simulink model "FloatingBall"  (R2024b)
settings: Solver=FixedStepAuto  StartTime=0.0  StopTime=inf  RelTol=1e-3  EnableMultiTasking=on
undefined symbols (not defined in the file or in its folder): Start
libraries: arduinolib x10, arduinoavrlib x2
settings Model: ExtModeTrigDuration=2  Creator=Tim  LastModifiedBy=Alexander
settings SolverCC: AutoInsertRateTranBlk=on
settings OptimizationCC: DefaultParameterBehavior=Inlined  EnhancedBackFolding=on  PassReuseOutputArgsAs=Individual arguments  ZeroExternalMemoryAtStartup=off  ZeroInternalMemoryAtStartup=off  MaxStackSize=64  OptimizeBlockOrder=speed  DifferentSizesBufferReuse=on  OptimizationCustomize=off  EfficientTunableParamExpr=on
settings DebuggingCC: MultiTaskDSMMsg=none  ParameterTunabilityLossMsg=error
settings HardwareCC: ProdBitPerInt=16  ProdBitPerPointer=16  ProdBitPerSizeT=16  ProdBitPerPtrDiffT=16  ProdLargestAtomicFloat=None  ProdWordSize=8  ProdHWDeviceType=Atmel->AVR
settings SFSimCC: MATLABDynamicMemAlloc=off
settings RTWCC: Description=Embedded Coder  SystemTargetFile=ert.tlc  HardwareBoard=Arduino Uno  TemplateMakefile=ert_default_tmf  Toolchain=Arduino AVR  BuildConfiguration=Faster Runs
settings CodeAppCC: ForceParamTrailComments=on  IgnoreCustomStorageClasses=off  OperatorAnnotations=on  SimulinkDataObjDesc=on  SFDataObjDesc=on  InsertBlockDesc=on
settings ERTTargetCC: SupportContinuousTime=on  SupportVariableSizeSignals=on  ExtModeTransport=3  ExtModeStaticAlloc=on  ExtModeAutomaticAllocSize=off  ExtModeStaticAllocSize=250  ExtModeMexFile=ext_xcp  ExtModeIntrfLevel=Level2 - Open

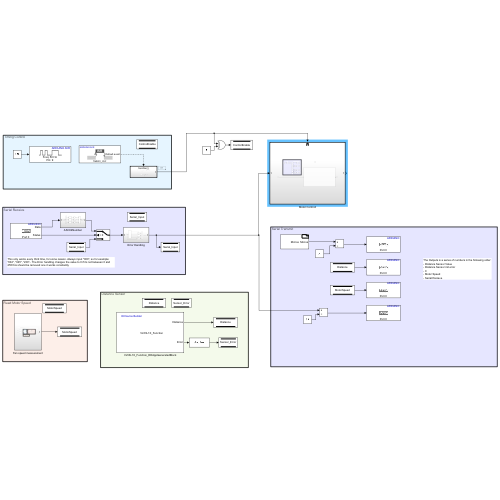
[thumbnail: Simulink's stored preview of the top-level diagram]
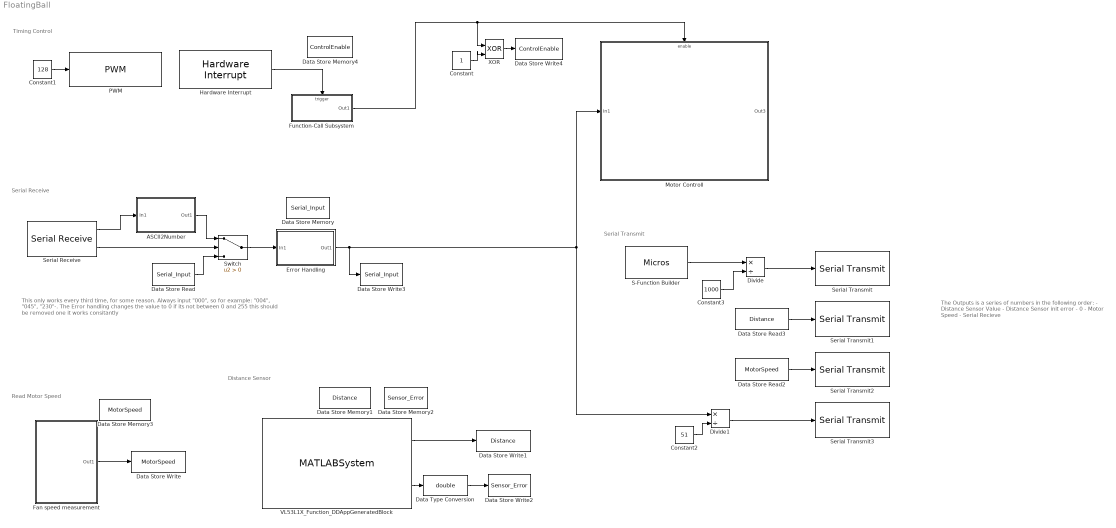
== system FloatingBall ==
  note: Timing Control
  note: Serial Receive
  note: This only works every third time, for some reason. Always input "000", so for example: "004", "045", "230"-. The Error handling changes the value to 0 if its not between 0 and 255 this should be removed one it works consitantly
  note: Read Motor Speed
  note: Distance Sensor
  note: The Outputs is a series of numbers in the following order:
      | - Distance Sensor Value
      | - Distance Sensor init error
      | - 0
      | - Motor Speed
      | - Serial Recieve
  note: Serial Transmit
  ASCII2Number : Subsystem
  Constant : Constant
  Constant1 : Constant  Value=128
  Constant2 : Constant  Value=51
  Constant3 : Constant  Value=1000
  Data Store Memory : DataStoreMemory  DataStoreName=Serial_Input  WriteAfterWriteMsg=warning  ShowAdditionalParam=off
  Data Store Memory1 : DataStoreMemory  DataStoreName=Distance  WriteAfterWriteMsg=warning  ShowAdditionalParam=off
  Data Store Memory2 : DataStoreMemory  DataStoreName=Sensor_Error  WriteAfterWriteMsg=warning  ShowAdditionalParam=off
  Data Store Memory3 : DataStoreMemory  DataStoreName=MotorSpeed  WriteAfterWriteMsg=warning  ShowAdditionalParam=off
  Data Store Memory4 : DataStoreMemory  DataStoreName=ControlEnable  WriteAfterWriteMsg=warning  ShowAdditionalParam=off
  Data Store Read : DataStoreRead  DataStoreName=Serial_Input  IndexOptions=Index vector (dialog)  Indices=1  OutputSizes=1
  Data Store Read2 : DataStoreRead  DataStoreName=MotorSpeed  IndexOptions=Index vector (dialog)  Indices=1  OutputSizes=1
  Data Store Read3 : DataStoreRead  DataStoreName=Distance  IndexOptions=Index vector (dialog)  Indices=1  OutputSizes=1
  Data Store Write : DataStoreWrite  DataStoreName=MotorSpeed  IndexOptions=Index vector (dialog)  Indices=1  OutputSizes=1
  Data Store Write1 : DataStoreWrite  DataStoreName=Distance  IndexOptions=Index vector (dialog)  Indices=1  OutputSizes=1
  Data Store Write2 : DataStoreWrite  DataStoreName=Sensor_Error  IndexOptions=Index vector (dialog)  Indices=1  OutputSizes=1
  Data Store Write3 : DataStoreWrite  DataStoreName=Serial_Input  IndexOptions=Index vector (dialog)  Indices=1  OutputSizes=1
  Data Store Write4 : DataStoreWrite  DataStoreName=ControlEnable  IndexOptions=Index vector (dialog)  Indices=1  OutputSizes=1
  Data Type Conversion : DataTypeConversion  OutDataTypeStr=double  SaturateOnIntegerOverflow=off  RndMeth=Floor
  Divide : Product  Inputs=*/
  Divide1 : Product  Inputs=*/
  Error Handling : Subsystem
  Fan speed measurement : Subsystem
  Function-Call Subsystem : Subsystem  TreatAsAtomicUnit=on
  Hardware Interrupt : arduinoavrlib/Hardware Interrupt  ISRGroup=Timer 1  ISRName=TIMER1_OVF  ISRNumber=7  EventsList={'on','Default event','1'}  SelectedEvents={'Default event'}  TaskPriority=8  DisablePreemption=on  ClearInterruptFlagsAtEndOfEvent=off  HardwareBoard=ARDUINO AVR
  Motor Controll : Subsystem
  PWM : arduinoavrlib/PWM  pinNumber=9  desiredFrequency=50  achievableFrequency=50  EnableCompareMatchInterrupt=off  EnableOverflowInterrupt=on
  S-Function Builder : S-Function  FunctionName=Micros  SFunctionModules=Micros_wrapper.c  SFunctionDeploymentMode=off  EnableBusSupport=off  mask(S-Function Builder){}
      mask help: Simulink:masks:SFunctionBuilder_MD
      mask init:
      | val = [[.9  0.75 0.75 1 1 .9 .9 1]',[1 1 0.75 0.75 .9 .9 1 .9]'];try , sys = get_param(gcb,'SfunBuilderFcnName');if isempty(sys), sys = get_param(gcb,'FunctionName'); end,catch, sys = get_param(gcb,'FunctionName'); end
      settings: CopyFcn=set_param(gcbh,'LinkStatus','none')  OpenFcn=sfunctionwizard(gcbh)
      mask Display:
      | plot(val(:,1),val(:,2))
      | disp(sys)
      | port_label('output',1,sprintf('%s', 'Micros'),'interpreter','tex')
  Serial Receive : arduinolib/Serial Receive  portNumber=0  DataType=uint8  blockPlatform=ARDUINO  TimeOut=0  MaxDataLength=2  isARMArch=off  DataLengthOption=Length via dialog  Datalength=3  Header=[]  Terminator=[]  SampleTime=0.02  ShowOutStatus=on
  Serial Transmit : arduinolib/Serial Transmit  portNumber=0  sendmode=print  label=;Start:  sendformat=Decimal  floatprecision=2  header=[]  terminator=[]  blockPlatform=ARDUINO
  Serial Transmit1 : arduinolib/Serial Transmit  portNumber=0  sendmode=print  label=;  sendformat=Decimal  floatprecision=1  header=[]  terminator=[]  blockPlatform=ARDUINO
  Serial Transmit2 : arduinolib/Serial Transmit  portNumber=0  sendmode=print  label=;  sendformat=Decimal  floatprecision=1  header=[]  terminator=[]  blockPlatform=ARDUINO
  Serial Transmit3 : arduinolib/Serial Transmit  portNumber=0  sendmode=print  label=;  sendformat=Decimal  floatprecision=2  header=[]  terminator=[]  blockPlatform=ARDUINO
  Switch : Switch  Criteria=u2 > Threshold  SaturateOnIntegerOverflow=off  InputSameDT=off
  VL53L1X_Function_DDAppGeneratedBlock : MATLABSystem  System=VL53L1X_Function  SampleTime=0.02
      mask Type: VL53L1X_Function
      mask Display:
      | color('white');plot([100,100,100,100]*1,[100,100,100,100]*1);plot([100,100,100,100]*0,[100,100,100,100]*0);color('blue');text(38, 92, 'IO Device Builder','horizontalAlignment', 'right');
      | color('black');text(52,50,' VL53L1X_Function','horizontalAlignment','center');
      | port_label('output',1,'Distance');port_label('output',2,'Error');
  XOR : Logic  Operator=XOR  IconShape=distinctive  AllPortsSameDT=off  OutDataTypeStr=boolean
  wires:
  Serial Receive/2 -> Switch/2
  Data Store Read/1 -> Switch/3
  Serial Receive/1 -> ASCII2Number/1(In1)
  ASCII2Number/1(Out1) -> Switch/1
  Switch/1 -> Error Handling/1(In1)
  Constant1/1 -> PWM/1
  Hardware Interrupt/1 -> Function-Call Subsystem/Trigger
  Fan speed measurement/1(Out1) -> Data Store Write/1
  VL53L1X_Function_DDAppGeneratedBlock/1 -> Data Store Write1/1
  VL53L1X_Function_DDAppGeneratedBlock/2 -> Data Type Conversion/1
  Data Type Conversion/1 -> Data Store Write2/1
  Function-Call Subsystem/1(Out1) -> Motor Controll/Enable, XOR/1
  Data Store Read2/1 -> Serial Transmit2/1
  Data Store Read3/1 -> Serial Transmit1/1
  S-Function Builder/1 -> Divide/1
  Constant3/1 -> Divide/2
  Divide/1 -> Serial Transmit/1
  Constant2/1 -> Divide1/2
  Divide1/1 -> Serial Transmit3/1
  Error Handling/1(Out1) -> Divide1/1, Motor Controll/1(In1), Data Store Write3/1
  XOR/1 -> Data Store Write4/1
  Constant/1 -> XOR/2

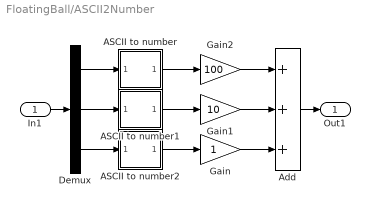
== system FloatingBall/ASCII2Number ==
  In1 : Inport
  ASCII to number : Subsystem
  ASCII to number1 : Subsystem
  ASCII to number2 : Subsystem
  Add : Sum  Inputs=+++
  Demux : Demux  Outputs=3
  Gain : Gain
  Gain1 : Gain  Gain=10
  Gain2 : Gain  Gain=100
  Out1 : Outport
  wires:
  Gain1/1 -> Add/2
  Gain2/1 -> Add/1
  Gain/1 -> Add/3
  Demux/1 -> ASCII to number/1(In1)
  ASCII to number2/1(Out1) -> Gain/1
  Demux/3 -> ASCII to number2/1(In1)
  ASCII to number/1(Out1) -> Gain2/1
  Demux/2 -> ASCII to number1/1(In1)
  ASCII to number1/1(Out1) -> Gain1/1
  Add/1 -> Out1/1
  In1/1 -> Demux/1

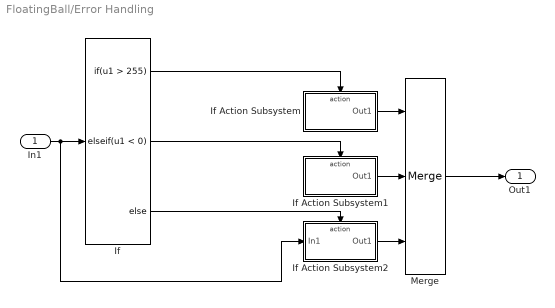
== system FloatingBall/Error Handling ==
  In1 : Inport
  If : If  IfExpression=u1 > 255  ElseIfExpressions=u1 < 0
  If Action Subsystem : Subsystem  TreatAsAtomicUnit=on
  If Action Subsystem1 : Subsystem  TreatAsAtomicUnit=on
  If Action Subsystem2 : Subsystem  TreatAsAtomicUnit=on
  Merge : Merge  Inputs=3
  Out1 : Outport
  wires:
  In1/1 -> If Action Subsystem2/1(In1), If/1
  If/1 -> If Action Subsystem/Action
  If/2 -> If Action Subsystem1/Action
  If/3 -> If Action Subsystem2/Action
  If Action Subsystem2/1(Out1) -> Merge/3
  If Action Subsystem1/1(Out1) -> Merge/2
  If Action Subsystem/1(Out1) -> Merge/1
  Merge/1 -> Out1/1

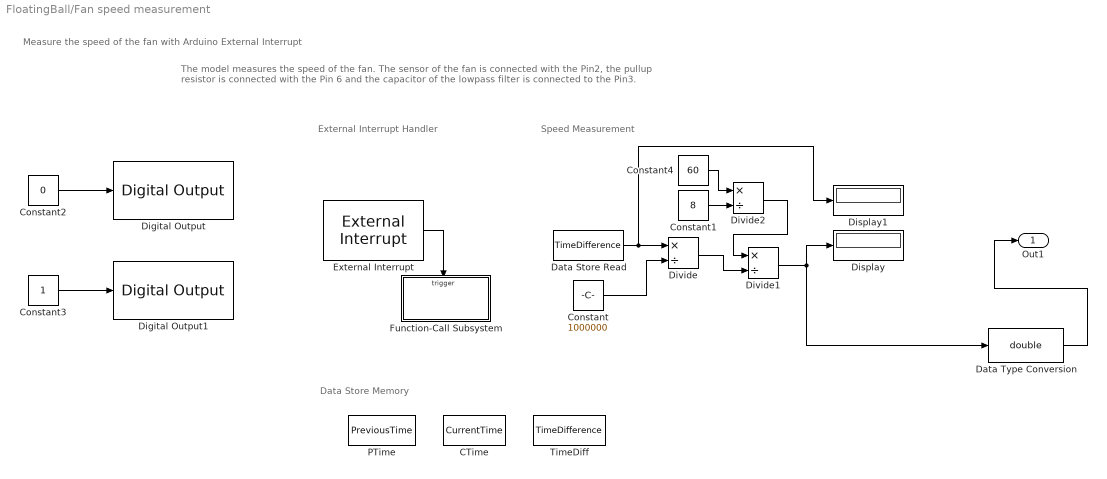
== system FloatingBall/Fan speed measurement ==
  note: External Interrupt Handler
  note: Speed Measurement
  note: Data Store Memory
  note: Measure the speed of the fan with Arduino External Interrupt
  note: The model measures the speed of the fan.
      | The sensor of the fan is connected with the Pin2, the pullup resistor is connected with the Pin 6 and
      | the capacitor of the lowpass filter is connected to the Pin3.
  CTime : DataStoreMemory  DataStoreName=CurrentTime  ShowAdditionalParam=off  OutDataTypeStr=uint32
  Constant : Constant  Value=1000000
  Constant1 : Constant  Value=8
  Constant2 : Constant  Value=0
  Constant3 : Constant
  Constant4 : Constant  Value=60
  Data Store Read : DataStoreRead  DataStoreName=TimeDifference  IndexOptions=Index vector (dialog)  Indices=1  OutputSizes=1
  Data Type Conversion : DataTypeConversion  OutDataTypeStr=double  SaturateOnIntegerOverflow=off  RndMeth=Floor
  Digital Output : arduinolib/Digital Output  pinNumber=3  Direction=output  blockPlatform=arduino
  Digital Output1 : arduinolib/Digital Output  pinNumber=6  Direction=output  blockPlatform=arduino
  Display : Display
  Display1 : Display
  Divide : Product  Inputs=*/
  Divide1 : Product  Inputs=*/
  Divide2 : Product  Inputs=*/
  External Interrupt : arduinolib/External Interrupt  Pin=2  PullUp=off  Mode=FALLING  InterruptSimulationInput=off
  Function-Call Subsystem : Subsystem  TreatAsAtomicUnit=on
  PTime : DataStoreMemory  DataStoreName=PreviousTime  ShowAdditionalParam=off  OutDataTypeStr=uint32
  TimeDiff : DataStoreMemory  DataStoreName=TimeDifference  ShowAdditionalParam=off  OutDataTypeStr=uint32
  Out1 : Outport
  wires:
  Divide/1 -> Divide1/2
  Constant/1 -> Divide/2
  External Interrupt/1 -> Function-Call Subsystem/Trigger
  Constant1/1 -> Divide2/2
  Data Store Read/1 -> Display1/1, Divide/1
  Constant3/1 -> Digital Output1/1
  Constant2/1 -> Digital Output/1
  Constant4/1 -> Divide2/1
  Data Type Conversion/1 -> Out1/1
  Divide2/1 -> Divide1/1
  Divide1/1 -> Display/1, Data Type Conversion/1

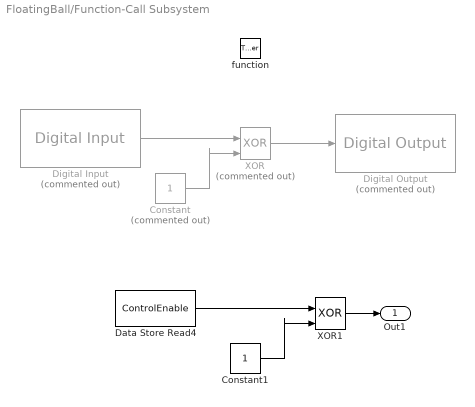
== system FloatingBall/Function-Call Subsystem ==
  function : TriggerPort  TriggerType=function-call  VariantControl=(inherit)
  Constant : Constant  Commented=on
  Constant1 : Constant
  Data Store Read4 : DataStoreRead  DataStoreName=ControlEnable  IndexOptions=Index vector (dialog)  Indices=1  OutputSizes=1
  Digital Input : arduinolib/Digital Input  Commented=on  pinNumber=12  mode=Default  Direction=input  SampleTime=-1  blockPlatform=arduino
  Digital Output : arduinolib/Digital Output  Commented=on  pinNumber=13  Direction=output  blockPlatform=arduino
  XOR : Logic  Commented=on  Operator=XOR  IconShape=distinctive  AllPortsSameDT=off  OutDataTypeStr=boolean
  XOR1 : Logic  Operator=XOR  IconShape=distinctive  AllPortsSameDT=off  OutDataTypeStr=boolean
  Out1 : Outport
  wires:
  Constant/1 -> XOR/2
  Digital Input/1 -> XOR/1
  XOR/1 -> Digital Output/1
  Constant1/1 -> XOR1/2
  Data Store Read4/1 -> XOR1/1
  XOR1/1 -> Out1/1

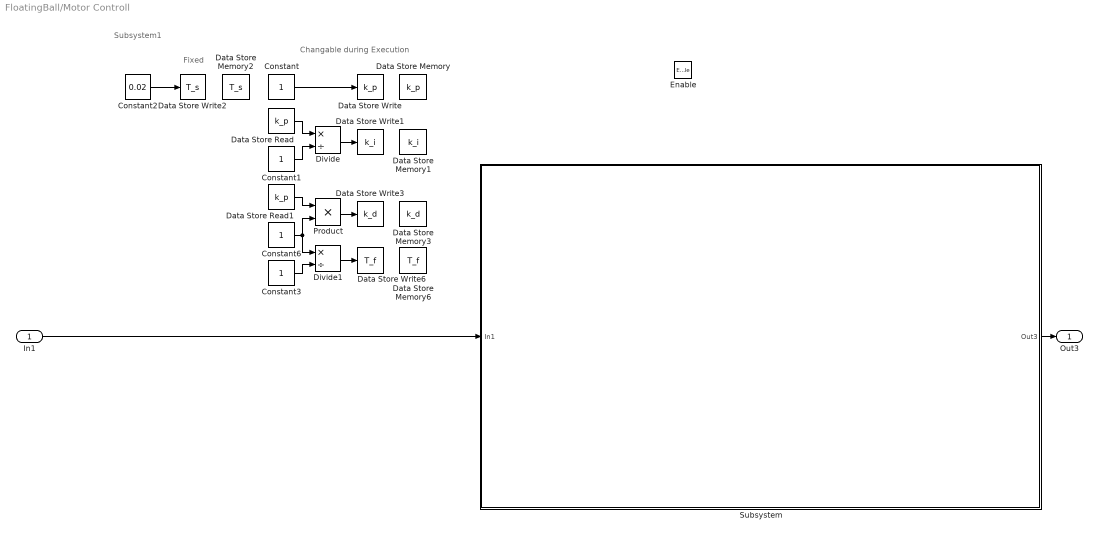
== system FloatingBall/Motor Controll ==
  note: Subsystem1
  note: Fixed
  note: Changable during Execution
  In1 : Inport
  Enable : EnablePort
  Constant{,1,3,6} (4 alike) : Constant
  Constant2 : Constant  Value=0.02
  Data Store Memory : DataStoreMemory  DataStoreName=k_p  WriteAfterWriteMsg=warning  ShowAdditionalParam=off
  Data Store Memory1 : DataStoreMemory  DataStoreName=k_i  WriteAfterWriteMsg=warning  ShowAdditionalParam=off
  Data Store Memory2 : DataStoreMemory  DataStoreName=T_s  WriteAfterWriteMsg=warning  ShowAdditionalParam=off
  Data Store Memory3 : DataStoreMemory  DataStoreName=k_d  WriteAfterWriteMsg=warning  ShowAdditionalParam=off
  Data Store Memory6 : DataStoreMemory  DataStoreName=T_f  WriteAfterWriteMsg=warning  ShowAdditionalParam=off
  Data Store Read : DataStoreRead  DataStoreName=k_p  IndexOptions=Index vector (dialog)  Indices=1  OutputSizes=1
  Data Store Read1 : DataStoreRead  DataStoreName=k_p  IndexOptions=Index vector (dialog)  Indices=1  OutputSizes=1
  Data Store Write : DataStoreWrite  DataStoreName=k_p  IndexOptions=Index vector (dialog)  Indices=1  OutputSizes=1
  Data Store Write1 : DataStoreWrite  DataStoreName=k_i  IndexOptions=Index vector (dialog)  Indices=1  OutputSizes=1
  Data Store Write2 : DataStoreWrite  DataStoreName=T_s  IndexOptions=Index vector (dialog)  Indices=1  OutputSizes=1
  Data Store Write3 : DataStoreWrite  DataStoreName=k_d  IndexOptions=Index vector (dialog)  Indices=1  OutputSizes=1
  Data Store Write6 : DataStoreWrite  DataStoreName=T_f  IndexOptions=Index vector (dialog)  Indices=1  OutputSizes=1
  Divide : Product  Inputs=*/
  Divide1 : Product  Inputs=*/
  Product : Product
  Subsystem : Subsystem
  Out3 : Outport
  wires:
  In1/1 -> Subsystem/1(In1)
  Subsystem/1(Out3) -> Out3/1
  Divide/1 -> Data Store Write1/1
  Data Store Read1/1 -> Product/1
  Data Store Read/1 -> Divide/1
  Product/1 -> Data Store Write3/1
  Constant2/1 -> Data Store Write2/1
  Constant1/1 -> Divide/2
  Constant/1 -> Data Store Write/1
  Divide1/1 -> Data Store Write6/1
  Constant3/1 -> Divide1/2
  Constant6/1 -> Divide1/1, Product/2

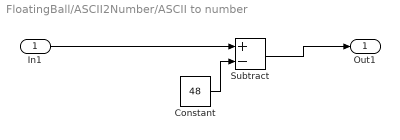
== system FloatingBall/ASCII2Number/ASCII to number ==
  In1 : Inport
  Constant : Constant  Value=48
  Subtract : Sum  Inputs=+-
  Out1 : Outport
  wires:
  In1/1 -> Subtract/1
  Constant/1 -> Subtract/2
  Subtract/1 -> Out1/1

== system FloatingBall/ASCII2Number/ASCII to number1 ==
  In1 : Inport
  Constant : Constant  Value=48
  Subtract : Sum  Inputs=+-
  Out1 : Outport
  wires:
  In1/1 -> Subtract/1
  Constant/1 -> Subtract/2
  Subtract/1 -> Out1/1

== system FloatingBall/ASCII2Number/ASCII to number2 ==
  In1 : Inport
  Constant : Constant  Value=48
  Subtract : Sum  Inputs=+-
  Out1 : Outport
  wires:
  In1/1 -> Subtract/1
  Constant/1 -> Subtract/2
  Subtract/1 -> Out1/1

== system FloatingBall/Error Handling/If Action Subsystem ==
  Action Port : ActionPort  ActionPortLabel=if(u1 > 255)
  Constant : Constant  Value=0
  Out1 : Outport
  wires:
  Constant/1 -> Out1/1

== system FloatingBall/Error Handling/If Action Subsystem1 ==
  Action Port : ActionPort  ActionPortLabel=elseif(u1 < 0)
  Constant : Constant  Value=0
  Out1 : Outport
  wires:
  Constant/1 -> Out1/1

== system FloatingBall/Error Handling/If Action Subsystem2 ==
  In1 : Inport
  Action Port : ActionPort  ActionPortLabel=else
  Out1 : Outport
  wires:
  In1/1 -> Out1/1

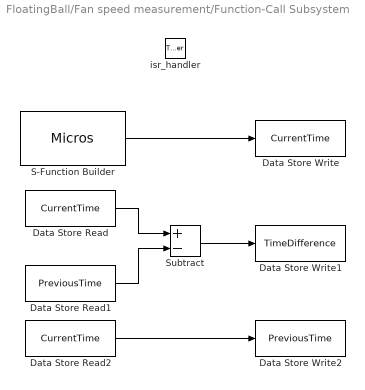
== system FloatingBall/Fan speed measurement/Function-Call Subsystem ==
  isr_handler : TriggerPort  TriggerType=function-call  VariantControl=Variant
  Data Store Read : DataStoreRead  DataStoreName=CurrentTime  IndexOptions=Index vector (dialog)  Indices=1  OutputSizes=1
  Data Store Read1 : DataStoreRead  DataStoreName=PreviousTime  IndexOptions=Index vector (dialog)  Indices=1  OutputSizes=1
  Data Store Read2 : DataStoreRead  DataStoreName=CurrentTime  IndexOptions=Index vector (dialog)  Indices=1  OutputSizes=1
  Data Store Write : DataStoreWrite  Priority=1  DataStoreName=CurrentTime  IndexOptions=Index vector (dialog)  Indices=1  OutputSizes=1
  Data Store Write1 : DataStoreWrite  Priority=2  DataStoreName=TimeDifference  IndexOptions=Index vector (dialog)  Indices=1  OutputSizes=1
  Data Store Write2 : DataStoreWrite  Priority=3  DataStoreName=PreviousTime  IndexOptions=Index vector (dialog)  Indices=1  OutputSizes=1
  S-Function Builder : S-Function  FunctionName=Micros  SFunctionModules=Micros_wrapper.c  SFunctionDeploymentMode=off  EnableBusSupport=off  mask(S-Function Builder){}
      mask help: Simulink:masks:SFunctionBuilder_MD
      mask init: same as FloatingBall/S-Function Builder
      settings: CopyFcn=set_param(gcbh,'LinkStatus','none')  OpenFcn=sfunctionwizard(gcbh)
      mask Display:
      | plot(val(:,1),val(:,2))
      | disp(sys)
      | port_label('output',1,sprintf('%s', 'Micros'),'interpreter','tex')
  Subtract : Sum  Inputs=+-
  wires:
  S-Function Builder/1 -> Data Store Write/1
  Data Store Read/1 -> Subtract/1
  Data Store Read1/1 -> Subtract/2
  Subtract/1 -> Data Store Write1/1
  Data Store Read2/1 -> Data Store Write2/1

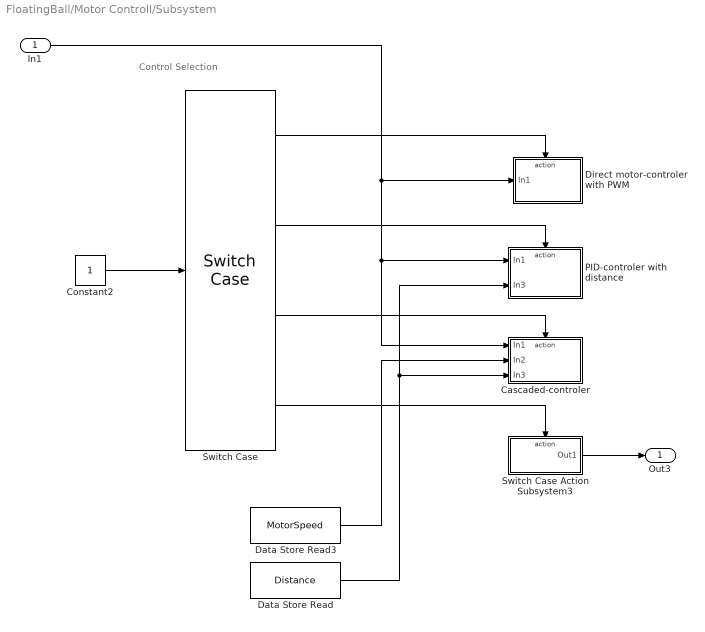
== system FloatingBall/Motor Controll/Subsystem ==
  note: Control Selection
  In1 : Inport
  Cascaded-controler : Subsystem  TreatAsAtomicUnit=on
  Constant2 : Constant
  Data Store Read : DataStoreRead  DataStoreName=Distance  IndexOptions=Index vector (dialog)  Indices=1  OutputSizes=1
  Data Store Read3 : DataStoreRead  DataStoreName=MotorSpeed  IndexOptions=Index vector (dialog)  Indices=1  OutputSizes=1
  Direct motor-controler with PWM : Subsystem  TreatAsAtomicUnit=on
  PID-controler with distance : Subsystem  TreatAsAtomicUnit=on
  Switch Case : SwitchCase  CaseConditions={1,2,3}
  Switch Case Action Subsystem3 : Subsystem  TreatAsAtomicUnit=on
  Out3 : Outport
  wires:
  Switch Case Action Subsystem3/1(Out1) -> Out3/1
  Switch Case/4 -> Switch Case Action Subsystem3/Action
  Data Store Read/1 -> Cascaded-controler/3(In3), PID-controler with distance/2(In3)
  In1/1 -> Direct motor-controler with PWM/1(In1), PID-controler with distance/1(In1), Cascaded-controler/1(In1)
  Switch Case/3 -> Cascaded-controler/Action
  Switch Case/2 -> PID-controler with distance/Action
  Switch Case/1 -> Direct motor-controler with PWM/Action
  Constant2/1 -> Switch Case/1
  Data Store Read3/1 -> Cascaded-controler/2(In2)

== system FloatingBall/Motor Controll/Subsystem/Cascaded-controler ==
  In1 : Inport
  In2 : Inport  Port=2
  In3 : Inport  Port=3
  Action Port : ActionPort  ActionPortLabel=case [ 3 ]:

== system FloatingBall/Motor Controll/Subsystem/Direct motor-controler with PWM ==
  note: Set Motor Speed
  In1 : Inport
  Action Port : ActionPort  ActionPortLabel=case [ 1 ]:
  Data Type Conversion2 : DataTypeConversion  OutDataTypeStr=uint8  SaturateOnIntegerOverflow=off  RndMeth=Floor
  MotorShield_Functions_DDAppGeneratedBlock : MATLABSystem  System=MotorShield_Functions  SampleTime=-1
      mask Type: MotorShield_Functions
      mask Display:
      | color('white');plot([100,100,100,100]*1,[100,100,100,100]*1);plot([100,100,100,100]*0,[100,100,100,100]*0);color('blue');text(38, 92, 'IO Device Builder','horizontalAlignment', 'right');
      | color('black');text(52,50,' MotorShield_Functions','horizontalAlignment','center');
      | port_label('input',1,'Speed');
  wires:
  Data Type Conversion2/1 -> MotorShield_Functions_DDAppGeneratedBlock/1
  In1/1 -> Data Type Conversion2/1

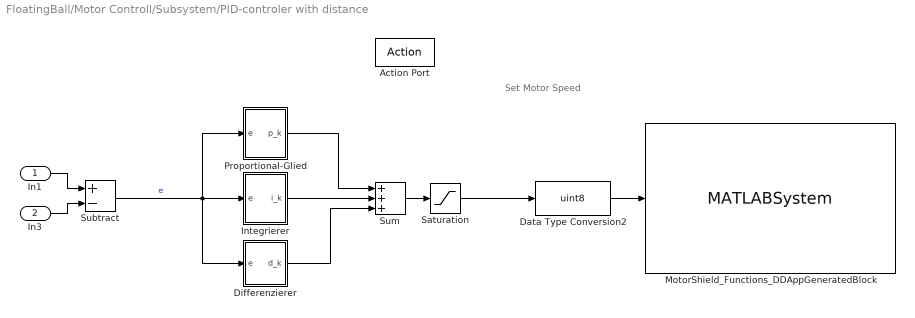
== system FloatingBall/Motor Controll/Subsystem/PID-controler with distance ==
  note: Set Motor Speed
  In1 : Inport
  In3 : Inport  Port=2
  Action Port : ActionPort  ActionPortLabel=case [ 2 ]:
  Data Type Conversion2 : DataTypeConversion  OutDataTypeStr=uint8  SaturateOnIntegerOverflow=off  RndMeth=Floor
  Differenzierer : Subsystem
  Integrierer : Subsystem
  MotorShield_Functions_DDAppGeneratedBlock : MATLABSystem  System=MotorShield_Functions  SampleTime=-1
      mask Type: MotorShield_Functions
      mask Display:
      | color('white');plot([100,100,100,100]*1,[100,100,100,100]*1);plot([100,100,100,100]*0,[100,100,100,100]*0);color('blue');text(38, 92, 'IO Device Builder','horizontalAlignment', 'right');
      | color('black');text(52,50,' MotorShield_Functions','horizontalAlignment','center');
      | port_label('input',1,'Speed');
  Proportional-Glied : Subsystem
  Saturation : Saturate  UpperLimit=255  LowerLimit=0
  Subtract : Sum  Inputs=+-
  Sum : Sum  Inputs=+++
  wires:
  Sum/1 -> Saturation/1
  Integrierer/1(i_k) -> Sum/2
  Proportional-Glied/1(p_k) -> Sum/1
  Differenzierer/1(d_k) -> Sum/3
  Subtract/1 -> Integrierer/1(e), Differenzierer/1(e), Proportional-Glied/1(e)  "e"
  Saturation/1 -> Data Type Conversion2/1
  Data Type Conversion2/1 -> MotorShield_Functions_DDAppGeneratedBlock/1
  In1/1 -> Subtract/1
  In3/1 -> Subtract/2

== system FloatingBall/Motor Controll/Subsystem/Switch Case Action Subsystem3 ==
  Action Port : ActionPort  ActionPortLabel=default:
  Constant : Constant
  Out1 : Outport
  wires:
  Constant/1 -> Out1/1

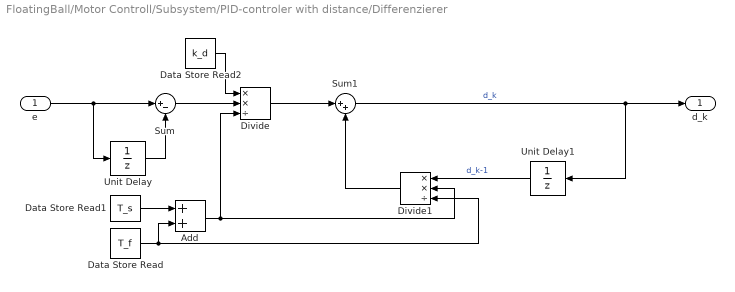
== system FloatingBall/Motor Controll/Subsystem/PID-controler with distance/Differenzierer ==
  e : Inport
  Add : Sum
  Data Store Read : DataStoreRead  DataStoreName=T_f  IndexOptions=Index vector (dialog)  Indices=1  OutputSizes=1
  Data Store Read1 : DataStoreRead  DataStoreName=T_s  IndexOptions=Index vector (dialog)  Indices=1  OutputSizes=1
  Data Store Read2 : DataStoreRead  DataStoreName=k_d  IndexOptions=Index vector (dialog)  Indices=1  OutputSizes=1
  Divide : Product  Inputs=**/
  Divide1 : Product  Inputs=**/
  Sum : Sum  Inputs=|+-
  Sum1 : Sum  Inputs=|++
  Unit Delay : UnitDelay  SampleTime=0.02  HasFrameUpgradeWarning=on
  Unit Delay1 : UnitDelay  SampleTime=0.02  HasFrameUpgradeWarning=on
  d_k : Outport
  wires:
  Sum1/1 -> Unit Delay1/1, d_k/1  "d_k"
  Divide/1 -> Sum1/1
  e/1 -> Unit Delay/1, Sum/1
  Sum/1 -> Divide/2
  Unit Delay/1 -> Sum/2
  Divide1/1 -> Sum1/2
  Unit Delay1/1 -> Divide1/1  "d_k-1"
  Add/1 -> Divide1/2, Divide/3
  Data Store Read1/1 -> Add/1
  Data Store Read/1 -> Add/2, Divide1/3
  Data Store Read2/1 -> Divide/1

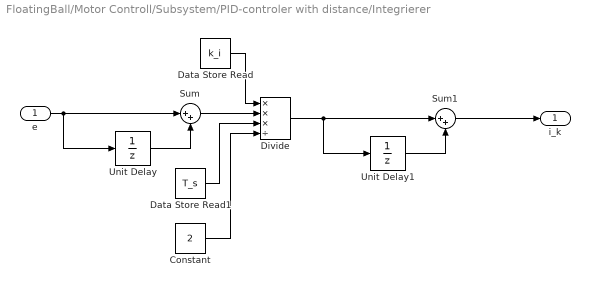
== system FloatingBall/Motor Controll/Subsystem/PID-controler with distance/Integrierer ==
  e : Inport
  Constant : Constant  Value=2
  Data Store Read : DataStoreRead  DataStoreName=k_i  IndexOptions=Index vector (dialog)  Indices=1  OutputSizes=1
  Data Store Read1 : DataStoreRead  DataStoreName=T_s  IndexOptions=Index vector (dialog)  Indices=1  OutputSizes=1
  Divide : Product  Inputs=***/
  Sum : Sum  Inputs=|++
  Sum1 : Sum  Inputs=|++
  Unit Delay : UnitDelay  SampleTime=0.02  HasFrameUpgradeWarning=on
  Unit Delay1 : UnitDelay  SampleTime=0.02  HasFrameUpgradeWarning=on
  i_k : Outport
  wires:
  Divide/1 -> Unit Delay1/1, Sum1/1
  Sum/1 -> Divide/2
  e/1 -> Sum/1, Unit Delay/1
  Sum1/1 -> i_k/1
  Unit Delay1/1 -> Sum1/2
  Data Store Read1/1 -> Divide/3
  Unit Delay/1 -> Sum/2
  Data Store Read/1 -> Divide/1
  Constant/1 -> Divide/4

== system FloatingBall/Motor Controll/Subsystem/PID-controler with distance/Proportional-Glied ==
  e : Inport
  Data Store Read : DataStoreRead  DataStoreName=k_p  IndexOptions=Index vector (dialog)  Indices=1  OutputSizes=1
  Product : Product
  p_k : Outport
  wires:
  Product/1 -> p_k/1  "p_k"
  e/1 -> Product/2
  Data Store Read/1 -> Product/1
